simulink model "target_drone"  (R2021a)
settings: Solver=VariableStepAuto  StartTime=0.0  StopTime=10000  RelTol=1e-3
settings Model: Creator=FJJ  LastModifiedBy=FJJ

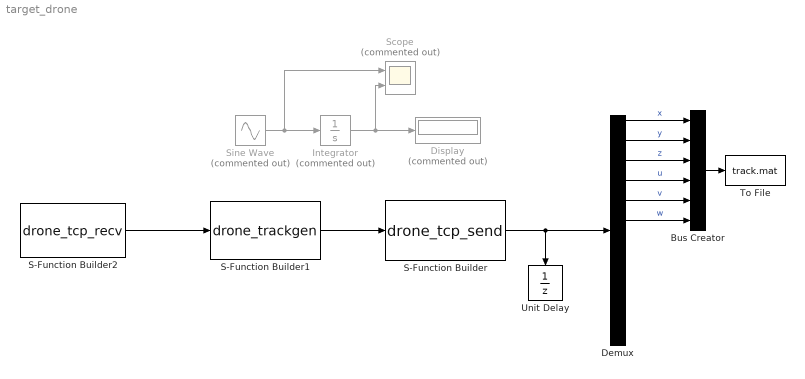
== system target_drone ==
  Bus Creator : BusCreator  Inputs=6
  Demux : Demux  Outputs=12
  Display : Display  Commented=on
  Integrator : Integrator  Commented=on
  S-Function Builder : S-Function  FunctionName=drone_tcp_send  Parameters=uint8([202,120,40,8]),int32(30608)  SFunctionModules=drone_tcp_send_wrapper  SFunctionDeploymentMode=off  EnableBusSupport=off  mask(S-Function Builder){}
      mask help: Simulink:masks:SFunctionBuilder_MD
      mask init:
      | val = [[.9  0.75 0.75 1 1 .9 .9 1]',[1 1 0.75 0.75 .9 .9 1 .9]'];try , sys = get_param(gcb,'SfunBuilderFcnName');if isempty(sys), sys = get_param(gcb,'FunctionName'); end,catch, sys = get_param(gcb,'FunctionName'); end
      settings: CopyFcn=set_param(gcbh,'LinkStatus','none')  OpenFcn=sfunctionwizard(gcbh)
      mask Display:
      | plot(val(:,1),val(:,2))
      | disp(sys)
      | port_label('input',1,'u0')
      | port_label('output',1,'y0')
  S-Function Builder1 : S-Function  FunctionName=drone_trackgen  SFunctionModules=drone_trackgen_wrapper  SFunctionDeploymentMode=off  EnableBusSupport=off  mask(S-Function Builder){}
      mask help: Simulink:masks:SFunctionBuilder_MD
      mask init: same as target_drone/S-Function Builder
      settings: CopyFcn=set_param(gcbh,'LinkStatus','none')  OpenFcn=sfunctionwizard(gcbh)
      mask Display:
      | plot(val(:,1),val(:,2))
      | disp(sys)
      | port_label('input',1,'in')
      | port_label('output',1,'out')
  S-Function Builder2 : S-Function  FunctionName=drone_tcp_recv  Parameters=uint8([202,120,40,8]),int32(30608)  SFunctionModules=drone_tcp_recv_wrapper  SFunctionDeploymentMode=off  EnableBusSupport=off  mask(S-Function Builder){}
      mask help: Simulink:masks:SFunctionBuilder_MD
      mask init: same as target_drone/S-Function Builder
      settings: CopyFcn=set_param(gcbh,'LinkStatus','none')  OpenFcn=sfunctionwizard(gcbh)
      mask Display:
      | plot(val(:,1),val(:,2))
      | disp(sys)
      | port_label('input',1,'u0')
      | port_label('output',1,'y0')
  Scope : Scope  Commented=on  NumInputPorts=2
  Sine Wave : Sin  Commented=on  SampleTime=0
  To File : ToFile  Filename=track.mat  SaveFormat=Timeseries
  Unit Delay : UnitDelay  InitialCondition=[100000, 0, 1000, 0, 0, 0, 0, 0, 0, 0, 0, 0]  SampleTime=-1  HasFrameUpgradeWarning=on
  wires:
  S-Function Builder1/1 -> S-Function Builder/1
  S-Function Builder/1 -> Unit Delay/1, Demux/1
  Demux/1 -> Bus Creator/1  "x"
  Demux/2 -> Bus Creator/2  "y"
  Demux/3 -> Bus Creator/3  "z"
  Demux/4 -> Bus Creator/4  "u"
  Demux/5 -> Bus Creator/5  "v"
  Demux/6 -> Bus Creator/6  "w"
  Bus Creator/1 -> To File/1
  Sine Wave/1 -> Integrator/1, Scope/1
  Integrator/1 -> Scope/2, Display/1
  S-Function Builder2/1 -> S-Function Builder1/1
